simulink library "NCS_Library"  (R2019a)
settings: Solver=VariableStepAuto  StartTime=0.0  StopTime=10.0  RelTol=1e-3
values from neighbouring files (symbols this model uses):
  A = 10    [Parameter.m]
  band = 100000000    [Parameter.m]
  BER = 0    [Parameter.m]
  c = 5000000    [Parameter.m]
  c1 = 4.33    [Parameter.m]
  c2 = 3.16    [Parameter.m]
  CAN2EthernetDelay = 0.000    (= 0)    [Parameter.m]
  cR = 1.5*10^-3    (= 0.0015)    [Parameter.m]
  cw = (cwE * 2 + cwM * (nW_ges-2))/nW_ges    (= 0.1475)    [Parameter.m]
  cwE = 0.35    [Parameter.m]
  cwM = 0.08    [Parameter.m]
  Cycle_Controller = 0    [Parameter.m]
  CyclePLC = 24/1000    (= 0.024)    [Parameter.m]
  d = 800000    [Parameter.m]
  Dr = 0.92    [Parameter.m]
  Ethernet2CANDelay = 0.005    [Parameter.m]
  F_konst = 70892    [Parameter.m]
  FA = 100000    [Parameter.m]
  FB_WB_max = 10000    [Parameter.m]
  FBel_an = iG*nG*F_KZmax*nBan*R_mR/(Dr/2)    (= 28197.4297239)    [Parameter.m]
  FBel_frei = iG*nG*F_KZmax*nBfrei*R_mW/(Dr/2)    (= 29270.6882948)    [Parameter.m]
  Fmaxdyn = 300000    [Parameter.m]
  g = 9.81    [Parameter.m]
  i = 0    [Parameter.m]
  J = 1/2*mA*(Dr/2)^2    (= 158.7)    [Parameter.m]
  k1 = 0.095    [Parameter.m]
  k2 = 9.26/3.6    (= 2.57222222222)    [Parameter.m]
  k3 = 4.63/3.6    (= 1.28611111111)    [Parameter.m]
  mges = 58000    [Parameter.m]
  mu = [mu1 mu2]    [Parameter.m]
  muBel1 = 0.42    [Parameter.m]
  muBel2 = 0.36    [Parameter.m]
  n = 0.001    [Parameter.m]
  n_Mg = 4    [Parameter.m]
  n_WB = 4    [Parameter.m]
  nA = 4    [Parameter.m]
  nBan = 2    [Parameter.m]
  nBfrei = 3    [Parameter.m]
  nM = 4    [Parameter.m]
  nW_an = 4    [Parameter.m]
  P_max = 8200000    [Parameter.m]
  Q = 10    [Parameter.m]
  r_reib = 600    [Parameter.m]
  rho = 1.08    [Parameter.m]
  rhoL = 1.225    [Parameter.m]
  Size = 8    [Parameter.m]
  slip = [s1 s2]    [Parameter.m]
  tol = 0.05    [Parameter.m]
  v00 = 100/3.6    (= 27.7777777778)    [Parameter.m]
  v_grenz = 60/3.6    (= 16.6666666667)    [Parameter.m]
  v_opt = 75/3.6    (= 20.8333333333)    [Parameter.m]
  W_opt = 0.5    [Parameter.m]
  WB = 1    [Parameter.m]
  y_opt = sqrt(W_opt)/((1+sqrt(W_opt))^2+W_opt)    [Parameter.m]
undefined symbols (not defined in the file or in its folder): BUSCapacity, CableLength, controlGate, D_dyn, D_mg, EnableBurst, EnableToF, entity, Entity_out, Gate, Gate_4, Gate_5, Gate_ACK, Gate_copy, Gate_RX, getData, gettime, I_dyn, I_mg, m, magnitude, P_dyn, P_mg, ReadAttributes, readdata, ReadData, ReadSize, sigbuilder_block, Timeout, ToB, ToF, v0, v_d, v_soll
libraries: simulink x176, $bdroot x102
(part 6 of 12)

== system NCS_Library/Network/ETB/Burst Device/Protocl Stack ==
  Signal : Inport
  Parameter : Inport  Port=2
  RxFromBus : Inport  Port=3
  Bus Creator1 : BusCreator  Inputs=13
  Bus Selector : BusSelector  OutputSignals=SDTv2,T_Tx,msgType
  CycleRx : EntityServer  InputPortMessageModes=m  OutputPortMessageModes=m  Capacity=inf  ServiceTimeValue=CycleRx
  CycleTx : EntityServer  InputPortMessageModes=m  OutputPortMessageModes=m  Capacity=inf  ServiceTimeValue=CycleTx
  Data Type Conversion{,1..6} (7 alike) : DataTypeConversion  OutDataTypeStr=double
  Detect Change : simulink/Logic and Bit Operations/Detect Change  vinit=0  OutDataTypeStr=boolean
  IP : $bdroot/Network/ETB/OSI Layers/IP  SystemSampleTime=-1
  MAC Controller : $bdroot/Network/ETB/OSI Layers/MAC Controller  SystemSampleTime=-1
  Multiply : Product
  SDTv2 : $bdroot/Network/ETB/OSI Layers/SDTv2  SystemSampleTime=-1
  TRDP PD : Subsystem
  TRDP Timeout : $bdroot/Network/ETB/OSI Layers/TRDP Timeout  SystemSampleTime=-1
  UDP Single-Port : $bdroot/Network/ETB/OSI Layers/UDP Single-Port  SystemSampleTime=-1
  Data : Outport
  Recorder : Outport  Port=2
  TxToBus : Outport  Port=3
  wires:
  TRDP Timeout/1 -> [Valid]
  [Valid] -> Multiply/1
  SDTv2/1 -> Multiply/2  "Data"
  Multiply/1 -> Bus Creator1/2, Data/1
  CycleTx/1 -> MAC Controller/1
  IP/4 -> CycleTx/1
  MAC Controller/1 -> CycleRx/1
  CycleRx/1 -> IP/3
  IP/3 -> Bus Creator1/10  "delay"
  IP/2 -> Data Type Conversion5/1
  TRDP PD/6(msgType_receive) -> Data Type Conversion2/1
  TRDP PD/5(#Receive) -> Data Type Conversion6/1, TRDP Timeout/1
  TRDP PD/4(msgType_transmit) -> Data Type Conversion/1
  TRDP PD/3(#Transmit) -> Data Type Conversion1/1
  SDTv2/3 -> Bus Creator1/4  "Phase"
  SDTv2/2 -> Data Type Conversion3/1
  [SDTv2] -> Bus Creator1/13  "SDTv2"
  RxFromBus/1 -> MAC Controller/3
  UDP Single-Port/2 -> IP/1
  IP/1 -> UDP Single-Port/2
  UDP Single-Port/1 -> TRDP PD/3(InFromUDP)
  MAC Controller/2 -> Bus Creator1/11  "#collision"
  Signal/1 -> Bus Creator1/1, SDTv2/1  "Signal"
  Parameter/1 -> Bus Selector/1, IP/2, MAC Controller/2, TRDP PD/2(Paramter)
  Data Type Conversion/1 -> Bus Creator1/6  "msgType_transmit"
  Bus Creator1/1 -> Recorder/1
  TRDP PD/7(OutToUDP) -> UDP Single-Port/1
  SDTv2/4 -> TRDP PD/1(InFromSDTv2)
  TRDP PD/2(TRM) -> SDTv2/6
  Bus Selector/2 -> SDTv2/3  "<T_Tx>"
  TRDP PD/1(OutToSDTv2) -> SDTv2/5
  Bus Selector/3 -> SDTv2/4  "<msgType>"
  MAC Controller/4 -> TxToBus/1
  MAC Controller/3 -> Detect Change/1  "Retry"
  Detect Change/1 -> Data Type Conversion4/1
  Bus Selector/1 -> [SDTv2], SDTv2/2  "<SDTv2>"
  Data Type Conversion1/1 -> Bus Creator1/5  "#Transmit"
  Data Type Conversion2/1 -> Bus Creator1/8  "msgType_receive"
  Data Type Conversion3/1 -> Bus Creator1/3  "SSC"
  Data Type Conversion4/1 -> Bus Creator1/12  "Retry"
  Data Type Conversion5/1 -> Bus Creator1/9  "#damaged"
  Data Type Conversion6/1 -> Bus Creator1/7  "#Receive"

== system NCS_Library/Network/ETB/Burst Device/Subsystem ==
  In1 : Inport
  Entity Input Switch : EntityInputSwitch  InputPortMessageModes=m,m,m,m,m,m,m,m,m,m  OutputPortMessageModes=m  NumberInputPorts=10
      settings: InputPortMap=u1,u2,u3,u4,u5,u6,u7,u8,u9,u10
  Entity Replicator : EntityReplicator  InputPortMessageModes=m  OutputPortMessageModes=m,m,m,m,m,m,m,m,m,m  NumberReplicas=9
      settings: OutputPortMap=o0,o1,o2,o3,o4,o5,o6,o7,o8,o9
  Out1 : Outport
  wires:
  Entity Replicator/10 -> Entity Input Switch/10
  Entity Replicator/9 -> Entity Input Switch/9
  Entity Replicator/8 -> Entity Input Switch/8
  Entity Replicator/7 -> Entity Input Switch/7
  Entity Replicator/6 -> Entity Input Switch/6
  Entity Replicator/5 -> Entity Input Switch/5
  Entity Replicator/4 -> Entity Input Switch/4
  Entity Replicator/3 -> Entity Input Switch/3
  Entity Replicator/2 -> Entity Input Switch/2
  Entity Replicator/1 -> Entity Input Switch/1
  Entity Input Switch/1 -> Out1/1
  In1/1 -> Entity Replicator/1

== system NCS_Library/Network/ETB/Burst Device/Subsystem1 ==
  In1 : Inport
  Constant : Constant  Value=0  OutDataTypeStr=uint16
  Constant1 : Constant  Value=0  OutDataTypeStr=uint16
  Mux : Mux  Inputs=3
  Out1 : Outport
  wires:
  Constant1/1 -> Mux/3
  Constant/1 -> Mux/2
  Mux/1 -> Out1/1
  In1/1 -> Mux/1

== system NCS_Library/Network/ETB/Burst Device/Subsystem2 ==
  In1 : Inport
  Constant : Constant  Value=0  OutDataTypeStr=uint16
  Constant1 : Constant  Value=0  OutDataTypeStr=uint16
  Display : Display
  Display1 : Display
  Mux : Mux  Inputs=3
  Out1 : Outport
  wires:
  In1/1 -> Display/1, Mux/1
  Mux/1 -> Display1/1, Out1/1
  Constant/1 -> Mux/2
  Constant1/1 -> Mux/3

== system NCS_Library/Network/ETB/Burst Device/Subsystem3 ==
  In1 : Inport
  Constant : Constant  Value=0  OutDataTypeStr=uint16
  Constant1 : Constant  Value=0  OutDataTypeStr=uint16
  Mux : Mux  Inputs=3
  Out1 : Outport
  wires:
  Constant1/1 -> Mux/3
  Constant/1 -> Mux/2
  Mux/1 -> Out1/1
  In1/1 -> Mux/1

== system NCS_Library/Network/ETB/Cable/Simulink Function ==
  Time : Inport
  BitError : TriggerPort  TriggerType=function-call  IsSimulinkFunction=on  FunctionName=BitError  FunctionVisibility=scoped  VariantControl=(inherit)
  Constant : Constant  Value=BER
  MATLAB Function : MATLAB Function  TreatAsAtomicUnit=on
  SubnetID1 : ArgIn  OutDataTypeStr=uint16  PortDimensions=[1 4]  ArgumentName=Source
  SEQ : ArgIn  Port=2  OutDataTypeStr=uint32  ArgumentName=SEQ
  CheckBit : ArgOut  DisableCoverage=on  OutDataTypeStr=uint8  ArgumentName=CheckBit
  wires:
  Constant/1 -> MATLAB Function/4(BER)
  Time/1 -> MATLAB Function/1(Time)
  SEQ/1 -> MATLAB Function/3(SEQ)
  MATLAB Function/1(CheckBit) -> CheckBit/1
  SubnetID1/1 -> MATLAB Function/2(Source)

== system NCS_Library/Network/ETB/Controller Interface/Parameter ==
  note: User defined Parameters
  Add : Sum  Inputs=+-
  Bus Creator : BusCreator  Inputs=8
  Constant : Constant  Value=Address  OutDataTypeStr=uint16
  Constant1 : Constant  Value=Actuators  OutDataTypeStr=uint16
  Constant10 : Constant  Value=msgType_2  OutDataTypeStr=uint16
  Constant11 : Constant  Value=msgType_3  OutDataTypeStr=uint16
  Constant12 : Constant  Value=msgType_4  OutDataTypeStr=uint16
  Constant13 : Constant  Value=SDTv2_2
  Constant14 : Constant  Value=SDTv2_3
  Constant15 : Constant  Value=SDTv2_4
  Constant16 : Constant  Value=[0 0 0 0]  OutDataTypeStr=uint16
  Constant2 : Constant  Value=Tx_1  OutDataTypeStr=double
  Constant3 : Constant  Value=msgType_1  OutDataTypeStr=uint16
  Constant4 : Constant  Value=SDTv2_1
  Constant5 : Constant
  Constant6 : Constant  OutDataTypeStr=uint16
  Constant7 : Constant  Value=Tx_2  OutDataTypeStr=double
  Constant8 : Constant  Value=Tx_3  OutDataTypeStr=double
  Constant9 : Constant  Value=Tx_4  OutDataTypeStr=double
  MATLAB Function : MATLAB Function  TreatAsAtomicUnit=on
  MATLAB Function1 : MATLAB Function  TreatAsAtomicUnit=on
  Mux : Mux
  Mux1 : Mux
  Subscribe : Constant  Value=Sensors  OutDataTypeStr=uint16
  Subsystem1 : $bdroot/Network/ETB/ED/User Interface/Subsystem2  SystemSampleTime=-1
  Out1 : Outport
  wires:
  Constant6/1 -> Bus Creator/5  "Port"
  Constant7/1 -> Mux/2
  Constant8/1 -> Mux/3
  Constant1/1 -> MATLAB Function1/1(Actuators)
  MATLAB Function1/2(Subscribe) -> Bus Creator/3  "Subscribe"
  Constant16/1 -> Bus Creator/4  "ReplyAddress"
  Constant5/1 -> Add/2
  Constant2/1 -> Mux/1
  Constant3/1 -> MATLAB Function/1(In1)
  Constant12/1 -> MATLAB Function/4(In4)
  Constant9/1 -> Mux/4
  Constant10/1 -> MATLAB Function/2(In2)
  Constant4/1 -> Mux1/1
  Constant11/1 -> MATLAB Function/3(In3)
  Constant13/1 -> Mux1/2
  Mux1/1 -> Add/1
  Constant14/1 -> Mux1/3
  Mux/1 -> Bus Creator/6  "T_Tx"
  Add/1 -> Bus Creator/8  "SDTv2"
  MATLAB Function/1(msgType) -> Bus Creator/7  "msgType"
  Subscribe/1 -> MATLAB Function1/2(Sensors)
  Constant15/1 -> Mux1/4
  Bus Creator/1 -> Out1/1
  MATLAB Function1/1(Destination) -> Bus Creator/2  "Destination"
  Constant/1 -> Subsystem1/1  "Address"
  Subsystem1/1 -> Bus Creator/1  "Address"

== system NCS_Library/Network/ETB/Controller Interface/Subsystem ==
  InFromController : Inport
  Parameter : Inport  Port=2
  RxFromBus : Inport  Port=3
  Application1 : $bdroot/Network/ETB/OSI Layers/Application  Port=1
  Application2 : $bdroot/Network/ETB/OSI Layers/Application  Port=2
  Application3 : $bdroot/Network/ETB/OSI Layers/Application  Port=3
  Application4 : $bdroot/Network/ETB/OSI Layers/Application  Port=4
  Bus Creator : BusCreator  Inputs=2
  Data Type Conversion : DataTypeConversion  OutDataTypeStr=double
  Mux Y_M : MATLAB Function  TreatAsAtomicUnit=on
  Parameter{1..4} (4 alike) : InportShadow  Port=2
  Transport Layers : Subsystem
  OutToController : Outport
  Recorder : Outport  Port=2
  TxToBus : Outport  Port=3
  wires:
  Parameter/1 -> Transport Layers/5(Parameter)
  RxFromBus/1 -> Transport Layers/6(RxFromBus)
  Transport Layers/7(TxToBus) -> TxToBus/1
  Parameter1/1 -> Application1/2
  Mux Y_M/1(Y_M) -> OutToController/1  "Y_M"
  Parameter2/1 -> Application2/2
  Parameter3/1 -> Application3/2
  Parameter4/1 -> Application4/2
  InFromController/1 -> Application1/1, Application2/1, Application4/1, Application3/1  "u_4"
  Application1/1 -> Mux Y_M/1(in1)  "y_M_1"
  Application2/1 -> Mux Y_M/2(in2)  "y_M_2"
  Application3/1 -> Mux Y_M/3(in3)  "y_M_3"
  Application4/1 -> Mux Y_M/4(in4)  "y_M_4"
  Transport Layers/1(OutToApplication4) -> Application4/3
  Application4/2 -> Transport Layers/1(InFromApplication4)
  Transport Layers/2(OutToApplication3) -> Application3/3
  Application3/2 -> Transport Layers/2(InFromApplication3)
  Transport Layers/3(OutToApplication2) -> Application2/3
  Application2/2 -> Transport Layers/3(InFromApplication2)
  Transport Layers/4(OutToApplication1) -> Application1/3
  Application1/2 -> Transport Layers/4(InFromApplication1)
  Transport Layers/5(Delay) -> Bus Creator/1  "Delay"
  Data Type Conversion/1 -> Bus Creator/2  "#damaged"
  Bus Creator/1 -> Recorder/1
  Transport Layers/6(#damaged) -> Data Type Conversion/1

== system NCS_Library/Network/ETB/ED/Protocol Stack ==
  Signal : Inport
  Parameter : Inport  Port=2
  RxFromBus : Inport  Port=3
  Bus Selector : BusSelector  OutputSignals=SDTv2,T_Tx,msgType
  CycleRx : EntityServer  InputPortMessageModes=m  OutputPortMessageModes=m  Capacity=inf  ServiceTimeValue=CycleRx
  CycleTx : EntityServer  InputPortMessageModes=m  OutputPortMessageModes=m  Capacity=inf  ServiceTimeValue=CycleTx  EntryAction=ReadSize(entity.Size);
  Display : Display
  IP : $bdroot/Network/ETB/OSI Layers/IP  SystemSampleTime=-1
  MAC Controller : $bdroot/Network/ETB/OSI Layers/MAC Controller  SystemSampleTime=-1
  Multiply : Product
  SDTv2 : $bdroot/Network/ETB/OSI Layers/SDTv2  SystemSampleTime=-1
  Signal1 : InportShadow
  Simulink Function : Subsystem  TreatAsAtomicUnit=on
  Subsystem : Subsystem
  TRDP PD : $bdroot/Network/ETB/OSI Layers/TRDP PD  SystemSampleTime=-1
  TRDP Timeout : $bdroot/Network/Applications/TRDP Timeout  SystemSampleTime=-1
  UDP Single-Port : $bdroot/Network/ETB/OSI Layers/UDP Single-Port  SystemSampleTime=-1
  Data : Outport
  Recorder : Outport  Port=2
  TxToBus : Outport  Port=3
  wires:
  Bus Selector/1 -> [SDTv2], SDTv2/2  "<SDTv2>"
  MAC Controller/4 -> TxToBus/1
  Bus Selector/3 -> SDTv2/4  "<msgType>"
  TRDP PD/1 -> SDTv2/5
  Bus Selector/2 -> SDTv2/3  "<T_Tx>"
  TRDP PD/2 -> SDTv2/6
  SDTv2/4 -> TRDP PD/1
  TRDP PD/7 -> UDP Single-Port/1
  Parameter/1 -> TRDP PD/3, MAC Controller/2, IP/2, Bus Selector/1
  Signal/1 -> SDTv2/1, Subsystem/1(Signal)  "Signal"
  UDP Single-Port/1 -> TRDP PD/4
  IP/1 -> UDP Single-Port/2
  UDP Single-Port/2 -> IP/1
  RxFromBus/1 -> MAC Controller/3
  CycleRx/1 -> IP/3
  MAC Controller/1 -> CycleRx/1
  IP/4 -> CycleTx/1
  CycleTx/1 -> MAC Controller/1
  Signal1/1 -> TRDP PD/2  "Signal"
  Multiply/1 -> Subsystem/2(Data), Data/1  "Data"
  SDTv2/1 -> Multiply/2  "Data"
  [Valid] -> Multiply/1
  SDTv2/2 -> Subsystem/3(In3)
  SDTv2/3 -> Subsystem/4(Phase)  "Phase"
  TRDP PD/3 -> Subsystem/5(In5)
  TRDP PD/4 -> Subsystem/6(In6)
  TRDP PD/5 -> TRDP Timeout/1, Subsystem/7(In7)
  TRDP PD/6 -> Subsystem/8(In8)
  IP/2 -> Subsystem/9(In9)
  IP/3 -> Subsystem/10(delay)  "delay"
  MAC Controller/2 -> Subsystem/11(#collision)  "#collision"
  MAC Controller/3 -> Subsystem/12(Retry)  "Retry"
  Subsystem/1(Out1) -> Recorder/1
  [SDTv2] -> Subsystem/13(SDTv2)  "SDTv2"
  TRDP Timeout/1 -> [Valid]
  Simulink Function/1(Out1) -> Display/1

== system NCS_Library/Network/ETB/ED/User Interface ==
  note: User defined Parameters
  Add : Sum  Inputs=+-
  Bus Creator : BusCreator  Inputs=8
  Constant : Constant  Value=Address  OutDataTypeStr=uint16
  Constant1 : Constant  Value=Destination  OutDataTypeStr=uint16
  Constant2 : Constant  Value=Tx  OutDataTypeStr=double
  Constant3 : Constant  Value=msgType  OutDataTypeStr=uint8
  Constant4 : Constant  Value=SDTv2  OutDataTypeStr=double
  Constant5 : Constant
  Constant6 : Constant  Value=Port  OutDataTypeStr=uint16
  Constant7 : Constant  Value=ReplyAddress  OutDataTypeStr=uint16
  MATLAB Function : MATLAB Function  TreatAsAtomicUnit=on
  MATLAB Function1 : MATLAB Function  TreatAsAtomicUnit=on
  Subscribe : Constant  Value=Subscribe  OutDataTypeStr=uint16
  Subsystem1 : $bdroot/Network/ETB/ED/User Interface/Subsystem2  SystemSampleTime=-1
  Subsystem2 : Subsystem
  Subsystem3 : $bdroot/Network/ETB/ED/User Interface/Subsystem2  SystemSampleTime=-1
  Parameter : Outport
  wires:
  Constant2/1 -> Bus Creator/6  "T_Tx"
  Constant3/1 -> MATLAB Function/1(u)
  MATLAB Function/1(msgType) -> Bus Creator/7  "msgType"
  Constant/1 -> Subsystem1/1
  Subsystem2/1(Out1) -> Bus Creator/2  "Destination"
  Constant7/1 -> Subsystem3/1
  Constant6/1 -> Bus Creator/5  "Port"
  Constant1/1 -> Subsystem2/1(In1)
  Subscribe/1 -> MATLAB Function1/1(u)
  Constant5/1 -> Add/2
  Constant4/1 -> Add/1
  Add/1 -> Bus Creator/8  "SDTv2"
  MATLAB Function1/1(y) -> Bus Creator/3  "Subscribe"
  Bus Creator/1 -> Parameter/1
  Subsystem1/1 -> Bus Creator/1  "Address"
  Subsystem3/1 -> Bus Creator/4  "ReplyAddress"

== system NCS_Library/Network/ETB/Ethernet_2-port_Switch/Buffer_fill Control ==
  In1 : Inport
  Compare To Constant : simulink/Logic and Bit Operations/Compare To Constant  relop=>=  const=floor(buffer_size/(2*1500))  OutDataTypeStr=boolean
  Constant : Constant
  Message Send : MessageSend  OutputPortMessageModes=m
      settings: InputPortMap=u1
  Sum : Sum  Inputs=|++
  Out1 : Outport
  wires:
  Message Send/1 -> Out1/1
  Sum/1 -> Message Send/1
  Constant/1 -> Sum/2
  Compare To Constant/1 -> Sum/1
  In1/1 -> Compare To Constant/1

== system NCS_Library/Network/ETB/Ethernet_2-port_Switch/Buffer_fill Control1 ==
  In1 : Inport
  Compare To Constant : simulink/Logic and Bit Operations/Compare To Constant  relop=>=  const=floor(buffer_size/(2*1500))  OutDataTypeStr=boolean
  Constant : Constant
  Message Send : MessageSend  OutputPortMessageModes=m
      settings: InputPortMap=u1
  Sum : Sum  Inputs=|++
  Out1 : Outport
  wires:
  Message Send/1 -> Out1/1
  Sum/1 -> Message Send/1
  Constant/1 -> Sum/2
  Compare To Constant/1 -> Sum/1
  In1/1 -> Compare To Constant/1

== system NCS_Library/Network/ETB/Ethernet_2-port_Switch/Determine Port_L//R ==
  gate_s : TriggerPort  TriggerType=function-call  IsSimulinkFunction=on  FunctionName=gate_s  FunctionVisibility=scoped  VariantControl=(inherit)
  Add : Sum
  Constant : Constant
  Constant1 : Constant  Value=addstore
  Data Store Read : DataStoreRead  DataStoreName=N
  Data Store Read1 : DataStoreRead  DataStoreName=S
  Data Store Write : DataStoreWrite  DataStoreName=S
  Data Type Conversion : DataTypeConversion  OutDataTypeStr=uint8
  Gain : Gain  Gain=1/band
  MATLAB Function1 : MATLAB Function  TreatAsAtomicUnit=on
  t1 : ArgIn  DisableCoverage=on  OutDataTypeStr=uint16  ArgumentName=Destination
  f1 : ArgIn  Port=2  OutDataTypeStr=uint16  ArgumentName=Source
  s : ArgIn  Port=3  ArgumentName=Size
  gate : ArgOut  OutDataTypeStr=uint8  ArgumentName=gate
  time : ArgOut  Port=2  ArgumentName=time
  wires:
  Constant/1 -> Add/2
  Gain/1 -> time/1
  s/1 -> Gain/1
  t1/1 -> MATLAB Function1/1(Destination)
  f1/1 -> MATLAB Function1/2(Source)
  MATLAB Function1/1(Anew) -> Data Store Write/1
  Data Store Read1/1 -> MATLAB Function1/3(A)
  Data Store Read/1 -> MATLAB Function1/4(B)
  Constant1/1 -> MATLAB Function1/5(maxn)
  MATLAB Function1/2(y) -> Add/1
  Add/1 -> Data Type Conversion/1
  Data Type Conversion/1 -> gate/1

== system NCS_Library/Network/ETB/Ethernet_2-port_Switch/Determine Port_N ==
  gate_n : TriggerPort  TriggerType=function-call  IsSimulinkFunction=on  FunctionName=gate_n  FunctionVisibility=scoped  VariantControl=(inherit)
  Add : Sum
  Constant : Constant
  Constant1 : Constant  Value=addstore
  Data Store Read : DataStoreRead  DataStoreName=N
  Data Store Read1 : DataStoreRead  DataStoreName=S
  Data Store Write : DataStoreWrite  DataStoreName=N
  Data Type Conversion : DataTypeConversion  OutDataTypeStr=uint8
  Gain : Gain  Gain=1/band
  MATLAB Function : MATLAB Function  TreatAsAtomicUnit=on
  t : ArgIn  DisableCoverage=on  OutDataTypeStr=uint16  ArgumentName=Destination
  f : ArgIn  Port=2  OutDataTypeStr=uint16  ArgumentName=Source
  s1 : ArgIn  Port=3  ArgumentName=Size
  gate : ArgOut  OutDataTypeStr=uint8  ArgumentName=gate
  time : ArgOut  Port=2  ArgumentName=time
  wires:
  f/1 -> MATLAB Function/2(Source)
  s1/1 -> Gain/1
  t/1 -> MATLAB Function/1(Destination)
  Add/1 -> Data Type Conversion/1
  Gain/1 -> time/1
  Data Store Read1/1 -> MATLAB Function/4(B)
  Data Store Read/1 -> MATLAB Function/3(A)
  Constant1/1 -> MATLAB Function/5(maxn)
  MATLAB Function/2(y) -> Add/1
  Constant/1 -> Add/2
  MATLAB Function/1(Anew) -> Data Store Write/1
  Data Type Conversion/1 -> gate/1

== system NCS_Library/Network/ETB/Ethernet_3-port_switch/Buffer_fill Control ==
  In1 : Inport
  Compare To Constant : simulink/Logic and Bit Operations/Compare To Constant  relop=>=  const=floor(buffer_size/(3*1500))  OutDataTypeStr=boolean
  Constant : Constant
  Message Send : MessageSend  OutputPortMessageModes=m
      settings: InputPortMap=u1
  Sum : Sum  Inputs=|++
  Out1 : Outport
  wires:
  In1/1 -> Compare To Constant/1
  Compare To Constant/1 -> Sum/1
  Constant/1 -> Sum/2
  Sum/1 -> Message Send/1
  Message Send/1 -> Out1/1

== system NCS_Library/Network/ETB/Ethernet_3-port_switch/Buffer_fill Control1 ==
  In1 : Inport
  Compare To Constant : simulink/Logic and Bit Operations/Compare To Constant  relop=>=  const=floor(buffer_size/(3*1500))  OutDataTypeStr=boolean
  Constant : Constant
  Message Send : MessageSend  OutputPortMessageModes=m
      settings: InputPortMap=u1
  Sum : Sum  Inputs=|++
  Out1 : Outport
  wires:
  In1/1 -> Compare To Constant/1
  Compare To Constant/1 -> Sum/1
  Constant/1 -> Sum/2
  Sum/1 -> Message Send/1
  Message Send/1 -> Out1/1

== system NCS_Library/Network/ETB/Ethernet_3-port_switch/Buffer_fill Control2 ==
  In1 : Inport
  Compare To Constant : simulink/Logic and Bit Operations/Compare To Constant  relop=>=  const=floor(buffer_size/(3*1500))  OutDataTypeStr=boolean
  Constant : Constant
  Message Send : MessageSend  OutputPortMessageModes=m
      settings: InputPortMap=u1
  Sum : Sum  Inputs=|++
  Out1 : Outport
  wires:
  In1/1 -> Compare To Constant/1
  Compare To Constant/1 -> Sum/1
  Constant/1 -> Sum/2
  Sum/1 -> Message Send/1
  Message Send/1 -> Out1/1

== system NCS_Library/Network/ETB/Ethernet_3-port_switch/Determine Port_L ==
  gate_l : TriggerPort  TriggerType=function-call  IsSimulinkFunction=on  FunctionName=gate_l  FunctionVisibility=scoped  VariantControl=(inherit)
  Add : Sum
  Constant : Constant
  Constant1 : Constant  Value=addstore
  Data Store Read : DataStoreRead  DataStoreName=N
  Data Store Read1 : DataStoreRead  DataStoreName=L
  Data Store Read2 : DataStoreRead  DataStoreName=R
  Data Store Write : DataStoreWrite  DataStoreName=L
  Data Type Conversion : DataTypeConversion  OutDataTypeStr=uint8
  Gain : Gain  Gain=1/band
  MATLAB Function : MATLAB Function  TreatAsAtomicUnit=on
  t~ : ArgIn  OutDataTypeStr=uint16  ArgumentName=Destination
  f~ : ArgIn  DisableCoverage=on  Port=2  OutDataTypeStr=uint16  ArgumentName=Source
  s : ArgIn  Port=3  ArgumentName=Size
  gate : ArgOut  OutDataTypeStr=uint8  ArgumentName=gate
  time : ArgOut  Port=2  ArgumentName=time
  wires:
  Gain/1 -> time/1
  Add/1 -> Data Type Conversion/1
  Constant/1 -> Add/2
  s/1 -> Gain/1
  MATLAB Function/1(Anew) -> Data Store Write/1
  MATLAB Function/2(y) -> Add/1
  t~/1 -> MATLAB Function/1(Destination)
  f~/1 -> MATLAB Function/2(Source)
  Data Store Read1/1 -> MATLAB Function/3(A)
  Data Store Read/1 -> MATLAB Function/4(B)
  Data Store Read2/1 -> MATLAB Function/5(C)
  Constant1/1 -> MATLAB Function/6(maxn)
  Data Type Conversion/1 -> gate/1

== system NCS_Library/Network/ETB/Ethernet_3-port_switch/Determine Port_N ==
  gate_n : TriggerPort  TriggerType=function-call  IsSimulinkFunction=on  FunctionName=gate_n  FunctionVisibility=scoped  VariantControl=(inherit)
  Add : Sum
  Constant : Constant
  Constant1 : Constant  Value=addstore
  Data Store Read : DataStoreRead  DataStoreName=N
  Data Store Read1 : DataStoreRead  DataStoreName=L
  Data Store Read2 : DataStoreRead  DataStoreName=R
  Data Store Write : DataStoreWrite  DataStoreName=N
  Data Type Conversion : DataTypeConversion  OutDataTypeStr=uint8
  Gain : Gain  Gain=1/band
  MATLAB Function : MATLAB Function  TreatAsAtomicUnit=on
  Destination : ArgIn  OutDataTypeStr=uint16  ArgumentName=Destination
  Source : ArgIn  DisableCoverage=on  Port=2  OutDataTypeStr=uint16  ArgumentName=Source
  Size : ArgIn  Port=3  ArgumentName=Size
  gate : ArgOut  OutDataTypeStr=uint8  ArgumentName=gate
  time : ArgOut  Port=2  ArgumentName=time
  wires:
  Constant/1 -> Add/2
  Gain/1 -> time/1
  Constant1/1 -> MATLAB Function/6(maxn)
  MATLAB Function/1(Anew) -> Data Store Write/1
  MATLAB Function/2(y) -> Add/1
  Data Store Read/1 -> MATLAB Function/3(A)
  Source/1 -> MATLAB Function/2(Source)
  Destination/1 -> MATLAB Function/1(Destination)
  Size/1 -> Gain/1
  Add/1 -> Data Type Conversion/1
  Data Type Conversion/1 -> gate/1
  Data Store Read1/1 -> MATLAB Function/4(B)
  Data Store Read2/1 -> MATLAB Function/5(C)

== system NCS_Library/Network/ETB/Ethernet_3-port_switch/Determine Port_R ==
  gate_r : TriggerPort  TriggerType=function-call  IsSimulinkFunction=on  FunctionName=gate_r  FunctionVisibility=scoped  VariantControl=(inherit)
  Add : Sum
  Constant : Constant
  Constant1 : Constant  Value=addstore
  Data Store Read : DataStoreRead  DataStoreName=N
  Data Store Read1 : DataStoreRead  DataStoreName=L
  Data Store Read2 : DataStoreRead  DataStoreName=R
  Data Store Write : DataStoreWrite  DataStoreName=R
  Data Type Conversion : DataTypeConversion  OutDataTypeStr=uint8
  Gain : Gain  Gain=1/band
  MATLAB Function : MATLAB Function  TreatAsAtomicUnit=on
  t~ : ArgIn  OutDataTypeStr=uint16  ArgumentName=Destination
  f~ : ArgIn  DisableCoverage=on  Port=2  OutDataTypeStr=uint16  ArgumentName=Source
  s : ArgIn  Port=3  ArgumentName=Size
  gate : ArgOut  OutDataTypeStr=uint8  ArgumentName=gate
  time : ArgOut  Port=2  ArgumentName=time
  wires:
  Constant/1 -> Add/2
  Gain/1 -> time/1
  Constant1/1 -> MATLAB Function/6(maxn)
  MATLAB Function/1(Anew) -> Data Store Write/1
  MATLAB Function/2(y) -> Add/1
  Data Store Read2/1 -> MATLAB Function/3(A)
  Data Store Read/1 -> MATLAB Function/4(B)
  Data Store Read1/1 -> MATLAB Function/5(C)
  f~/1 -> MATLAB Function/2(Source)
  t~/1 -> MATLAB Function/1(Destination)
  s/1 -> Gain/1
  Add/1 -> Data Type Conversion/1
  Data Type Conversion/1 -> gate/1

== system NCS_Library/Network/ETB/OSI Layers/Application ==
  InFromController : Inport
  Paramter : Inport  Port=2
  InFromUDP : Inport  Port=3
  Edit Paramter : Subsystem
  Entity Output Switch : EntityOutputSwitch  InputPortMessageModes=m  OutputPortMessageModes=m,m  SwitchingCriterion=From attribute  SwitchAttributeName=Route
  Entity Server : EntityServer  InputPortMessageModes=m  OutputPortMessageModes=m  Capacity=1  ServiceTimeValue=0  EntryAction=entity.Route = Sort(entity.msgType);
  Receive Sensor Data : Subsystem
  Simulink Function : Subsystem  TreatAsAtomicUnit=on
  Transmit Actuator Data : Subsystem
  UDP_Port : Constant  Value=Port  OutDataTypeStr=uint16
  OutToController : Outport
  OutToUDP : Outport  Port=2
  wires:
  UDP_Port/1 -> Edit Paramter/1(UDP_Port)
  Receive Sensor Data/1(OutToController) -> OutToController/1  "y_M"
  Paramter/1 -> Edit Paramter/2(Parameter)
  Edit Paramter/1(Parameter_edited) -> Receive Sensor Data/1(Parameter), Transmit Actuator Data/3(Parameter)
  InFromUDP/1 -> Entity Server/1
  Transmit Actuator Data/1(OutToUDP) -> OutToUDP/1
  InFromController/1 -> Transmit Actuator Data/1(InFromController)  "u"
  Entity Server/1 -> Entity Output Switch/1
  Entity Output Switch/1 -> Receive Sensor Data/2(InFromUDP)  "Push by Sensor"
  Entity Output Switch/2 -> Transmit Actuator Data/2(InFromUDP)  "Pull Request by Actuator"

== system NCS_Library/Network/ETB/OSI Layers/IP ==
  note: Get Delay
  note: Addressing
  note: Receive
  note: Transmit
  note: Check Sum
  InFromUDP : Inport
  Paramter : Inport  Port=2
  InFromMAC : Inport  Port=3
  Add : Sum  Inputs=+-
  Bus Selector : BusSelector  OutputSignals=Address,Subscribe
  Clock : Clock
  Detect Change2 : simulink/Logic and Bit Operations/Detect Change  vinit=0  OutDataTypeStr=boolean
  Display : Display
  Display1 : Display
  Entity Output Switch : EntityOutputSwitch  InputPortMessageModes=m  OutputPortMessageModes=m,m  SwitchingCriterion=From attribute  SwitchAttributeName=CheckBit
  Entity Output Switch1 : EntityOutputSwitch  InputPortMessageModes=m  OutputPortMessageModes=m,m  SwitchingCriterion=From attribute  SwitchAttributeName=Route
  Entity Server : EntityServer  InputPortMessageModes=m  OutputPortMessageModes=m  Capacity=1  ServiceTimeValue=0  EntryAction=[ entity.Timestamp, entity.MACDestination, entity.MACSource ] = SetAttributes(entity.Destination, entity.Source);
  Entity Server1 : EntityServer  InputPortMessageModes=m  OutputPortMessageModes=n,m  Capacity=1  ServiceTimeValue=0  EntryAction=|  NumberEntitiesDeparted=on
      | entity.Route = getAttributes(entity.Timestamp, entity.Source, entity.Destination);
      | entity.CheckBit = entity.CheckBit+uint8(1);
      settings: OutputPortMap=o0,o9
  Entity Server2 : EntityServer  InputPortMessageModes=m  OutputPortMessageModes=n,m  Capacity=1  ServiceTimeValue=0  NumberEntitiesDeparted=on
      settings: OutputPortMap=o0,o9
  Entity Terminator : EntityTerminator  InputPortMessageModes=m  NumberEntitiesArrived=on
      settings: OutputPortMap=o0
  Entity Terminator1 : EntityTerminator  InputPortMessageModes=m  NumberEntitiesArrived=on
      settings: OutputPortMap=o0
  Simulink Function : Subsystem  TreatAsAtomicUnit=on
  Simulink Function1 : Subsystem  TreatAsAtomicUnit=on
  Subsystem : Subsystem
  OutToUDP : Outport
  #damaged : Outport  Port=2
  DELAY : Outport  Port=3
  OutToMAC : Outport  Port=4
  wires:
  InFromUDP/1 -> Entity Server/1
  Entity Server/1 -> OutToMAC/1
  InFromMAC/1 -> Entity Server1/1
  Entity Output Switch/1 -> Entity Terminator/1
  Entity Terminator/1 -> #damaged/1
  Clock/1 -> Simulink Function/1(time), [Time]
  Simulink Function1/1(Timestamp) -> Add/2
  Detect Change2/1 -> Subsystem/Enable
  Subsystem/1(DELAY) -> DELAY/1
  Add/1 -> Subsystem/1(delay)
  [Time] -> Add/1
  Entity Output Switch1/2 -> Entity Terminator1/1
  Entity Server1/2 -> Entity Output Switch1/1
  Entity Output Switch1/1 -> Entity Output Switch/1
  Entity Output Switch/2 -> Entity Server2/1
  Entity Server2/2 -> OutToUDP/1
  Entity Server2/1 -> Detect Change2/1
  Entity Server1/1 -> Display/1
  Bus Selector/1 -> Simulink Function1/1(Address)  "<Address>"
  Bus Selector/2 -> Simulink Function1/2(SN)  "<Subscribe>"
  Paramter/1 -> Bus Selector/1
  Entity Terminator1/1 -> Display1/1
  Simulink Function1/2(Source) -> Subsystem/2(Source)
  Simulink Function1/3(Destination) -> Subsystem/3(Destination)

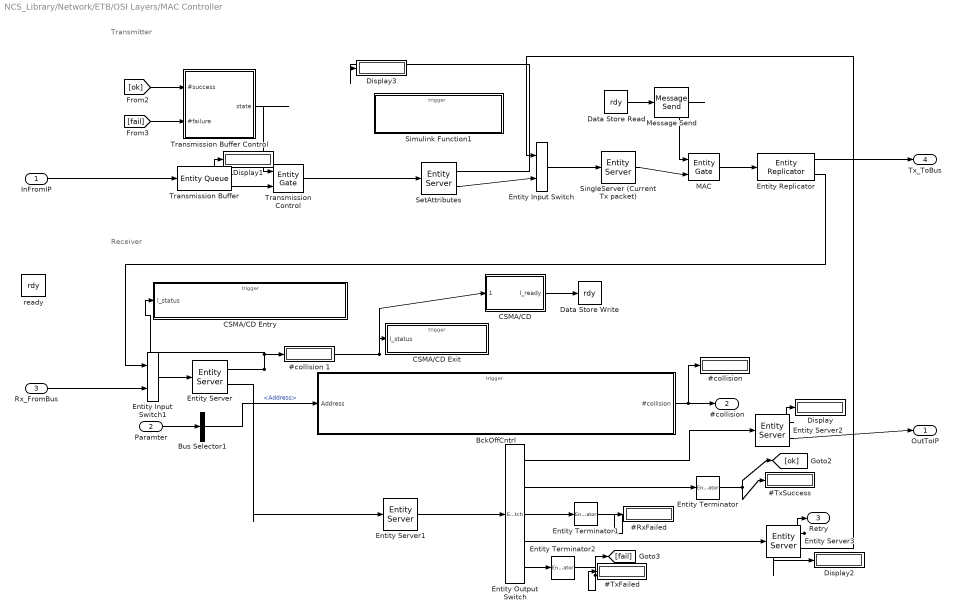
== system NCS_Library/Network/ETB/OSI Layers/MAC Controller ==
  note: Transmitter
  note: Receiver
  InFromIP : Inport
  Paramter : Inport  Port=2
  Rx_FromBus : Inport  Port=3
  #RxFailed : Display
  #TxFailed : Display
  #TxSuccess : Display
  "#collision " : Display
  #collision 1 : Display
  BckOffCntrl : Subsystem  TreatAsAtomicUnit=on
  Bus Selector1 : BusSelector  OutputSignals=Address
  CSMA/CD : Subsystem  TreatAsAtomicUnit=on
  CSMA/CD Entry : Subsystem  TreatAsAtomicUnit=on
  CSMA/CD Exit : Subsystem  TreatAsAtomicUnit=on
  Data Store Read : DataStoreRead  DataStoreName=rdy
  Data Store Write : DataStoreWrite  DataStoreName=rdy
  Display{,1..3} (4 alike) : Display
  Entity Input Switch : EntityInputSwitch  InputPortMessageModes=m,m  OutputPortMessageModes=m
  Entity Input Switch1 : EntityInputSwitch  InputPortMessageModes=m,m  OutputPortMessageModes=m
  Entity Output Switch : EntityOutputSwitch  InputPortMessageModes=m  OutputPortMessageModes=m,m,m,m,m  NumberOutputPorts=5  SwitchingCriterion=From attribute  SwitchAttributeName=Route
      settings: OutputPortMap=o0,o1,o2,o3,o4
  Entity Replicator : EntityReplicator  InputPortMessageModes=m  OutputPortMessageModes=m,m
  Entity Server : EntityServer  InputPortMessageModes=m  OutputPortMessageModes=n,m  Capacity=1000  ServiceTimeSource=Attribute  EntryAction=entity.ServiceTime = SetServiceTime(entity.Size);  NumberEntitiesInBlock=on
      settings: OutputPortMap=o1,o9
  Entity Server1 : EntityServer  InputPortMessageModes=m  OutputPortMessageModes=m  Capacity=1  ServiceTimeValue=0  EntryAction=[entity.Route,entity.NumCollision, entity.BckOffTime]=bckoffctrl(entity.NumCollision, entity.Collision, entity.MACSource, entity.MACDestination, entity.SEQ, entity.ServiceTime);
  Entity Server2 : EntityServer  InputPortMessageModes=m  OutputPortMessageModes=n,m  Capacity=1  ServiceTimeValue=0  NumberEntitiesDeparted=on
      settings: OutputPortMap=o0,o9
  Entity Server3 : EntityServer  InputPortMessageModes=m  OutputPortMessageModes=n,m  Capacity=1  ServiceTimeValue=0  NumberEntitiesDeparted=on
      settings: OutputPortMap=o0,o9
  Entity Terminator : EntityTerminator  InputPortMessageModes=m  NumberEntitiesArrived=on
      settings: OutputPortMap=o0
  Entity Terminator1 : EntityTerminator  InputPortMessageModes=m  NumberEntitiesArrived=on
      settings: OutputPortMap=o0
  Entity Terminator2 : EntityTerminator  InputPortMessageModes=m  NumberEntitiesArrived=on
      settings: OutputPortMap=o0
  MAC : EntityGate  InputPortMessageModes=m,m  OutputPortMessageModes=m
  Message Send : MessageSend  OutputPortMessageModes=m
      settings: InputPortMap=u1
  SetAttributes : EntityServer  InputPortMessageModes=m  OutputPortMessageModes=n,m  Capacity=1  ServiceTimeValue=0  EntryAction=|  NumberEntitiesDeparted=on
      | entity.ServiceTime = SetServiceTime(entity.Size);
      | % Init
      | entity.NumCollision=uint8(0);
      | entity.BckOffTime=0;
      settings: OutputPortMap=o0,o9
  Simulink Function1 : Subsystem  TreatAsAtomicUnit=on
  SingleServer (Current Tx packet) : EntityServer  InputPortMessageModes=m  OutputPortMessageModes=m  Capacity=1  ServiceTimeSource=Attribute  ServiceTimeValue=0  ServiceTimeAttributeName=BckOffTime  EntryAction=entity.Collision = uint8(0);
  Transmission Buffer : EntityQueue  InputPortMessageModes=m  OutputPortMessageModes=n,m  Capacity=100  NumberEntitiesInBlock=on
      settings: OutputPortMap=o1,o5
  Transmission Buffer Control : Subsystem
  Transmission Control : EntityGate  InputPortMessageModes=m,m  OutputPortMessageModes=m  OperatingMode=Release gate  OpenGateAtSimulationStart=on
  ready : DataStoreMemory  DataStoreName=rdy  ReadBeforeWriteMsg=warning  WriteAfterWriteMsg=warning  WriteAfterReadMsg=warning  InitialValue=1  ShowAdditionalParam=off
  OutToIP : Outport
  #collision : Outport  Port=2
  Retry : Outport  Port=3
  Tx_ToBus : Outport  Port=4
  wires:
  CSMA/CD/1(l_ready) -> Data Store Write/1
  Transmission Control/1 -> SetAttributes/1
  Entity Output Switch/2 -> Entity Terminator/1
  Data Store Read/1 -> Message Send/1
  Message Send/1 -> MAC/1
  Entity Output Switch/3 -> Entity Terminator1/1
  Entity Server1/1 -> Entity Output Switch/1
  SetAttributes/2 -> Entity Input Switch/2
  MAC/1 -> Entity Replicator/1
  Entity Input Switch1/1 -> Entity Server/1
  Entity Server/1 -> #collision 1/1, CSMA/CD Entry/1(l_status), CSMA/CD/1(l_status), CSMA/CD Exit/1(l_status)
  Entity Server/2 -> Entity Server1/1
  SingleServer (Current Tx packet)/1 -> MAC/2
  Entity Terminator1/1 -> #RxFailed/1
  Entity Input Switch/1 -> SingleServer (Current Tx packet)/1
  InFromIP/1 -> Transmission Buffer/1
  [ok] -> Transmission Buffer Control/1(#success)
  Transmission Buffer Control/1(state) -> Transmission Control/1
  [fail] -> Transmission Buffer Control/2(#failure)
  Transmission Buffer/2 -> Transmission Control/2
  Entity Output Switch/1 -> Entity Server2/1
  Entity Replicator/1 -> Tx_ToBus/1
  Entity Output Switch/5 -> Entity Terminator2/1
  Entity Replicator/2 -> Entity Input Switch1/1
  BckOffCntrl/1(#collision) -> #collision/1, "#collision "/1
  Rx_FromBus/1 -> Entity Input Switch1/2
  SetAttributes/1 -> Display3/1
  Paramter/1 -> Bus Selector1/1
  Bus Selector1/1 -> BckOffCntrl/1(Address)  "<Address>"
  Entity Server2/2 -> OutToIP/1
  Entity Terminator/1 -> [ok], #TxSuccess/1
  Entity Server2/1 -> Display/1
  Entity Output Switch/4 -> Entity Server3/1
  Entity Server3/2 -> Entity Input Switch/1
  Entity Server3/1 -> Retry/1, Display2/1
  Transmission Buffer/1 -> Display1/1
  Entity Terminator2/1 -> [fail], #TxFailed/1

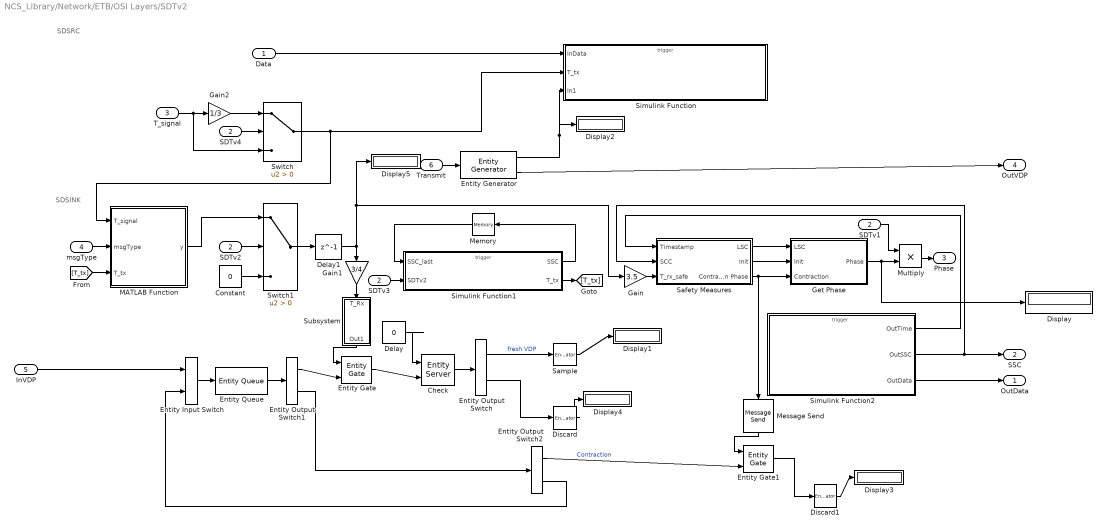
== system NCS_Library/Network/ETB/OSI Layers/SDTv2 ==
  note: SDSINK
  note: SDSRC
  Data : Inport
  SDTv2 : Inport  Port=2
  T_signal : Inport  Port=3
  msgType : Inport  Port=4
  InVDP : Inport  Port=5
  Transmit : Inport  Port=6
  Check : EntityServer  InputPortMessageModes=n,m  OutputPortMessageModes=m  Capacity=1  ServiceTimeSource=Signal port  ServiceTimeValue=0  EntryAction=[entity.Route] = Check(entity.SSC,entity.T_tx);
      settings: InputPortMap=u0,u2
  Constant : Constant  Value=0
  Delay : Constant  Value=0
  Delay1 : Delay  DelayLength=1
  Discard : EntityTerminator  InputPortMessageModes=m  NumberEntitiesArrived=on
      settings: OutputPortMap=o0
  Discard1 : EntityTerminator  InputPortMessageModes=m  NumberEntitiesArrived=on
      settings: OutputPortMap=o0
  Display{,1..5} (6 alike) : Display
  Entity Input Switch : EntityInputSwitch  InputPortMessageModes=m,m  OutputPortMessageModes=m
  Entity Output Switch : EntityOutputSwitch  InputPortMessageModes=m  OutputPortMessageModes=m,m  SwitchingCriterion=From attribute  SwitchAttributeName=Route
  Entity Output Switch1 : EntityOutputSwitch  InputPortMessageModes=m  OutputPortMessageModes=m,m  SwitchAttributeName=Attribute1
  Entity Output Switch2 : EntityOutputSwitch  InputPortMessageModes=m  OutputPortMessageModes=m,m  SwitchAttributeName=Attribute1
  Entity Gate : EntityGate  InputPortMessageModes=m,m  OutputPortMessageModes=m
  Entity Gate1 : EntityGate  InputPortMessageModes=m,m  OutputPortMessageModes=m  OpenGateAtSimulationStart=on
  Entity Generator : EntityGenerator  InputPortMessageModes=m  OutputPortMessageModes=n,m  GenerationMethod=Event-based  TimeSource=Signal port  GenerateAction=[ entity.SSC, entity.Data, entity.T_tx, entity.Size ] = SetAttributes();  NumberEntitiesDeparted=on  EntityType=Bus object  EntityTypeName=Ethernet_Entity
      settings: InputPortMap=u0  OutputPortMap=o0,o3
  Entity Queue : EntityQueue  InputPortMessageModes=m  OutputPortMessageModes=m
      settings: OutputPortMap=o5
  Gain : Gain  Gain=3.5
  Gain1 : Gain  Gain=3/4
  Gain2 : Gain  Gain=1/3
  Get Phase : Subsystem
  MATLAB Function : MATLAB Function  TreatAsAtomicUnit=on
  Memory : Memory  InheritSampleTime=on
  Message Send : MessageSend  OutputPortMessageModes=m
      settings: InputPortMap=u1
  Multiply : Product
  SDTv1 : InportShadow  Port=2
  SDTv3 : InportShadow  Port=2
  SDTv4 : InportShadow  Port=2
  Safety Measures : Subsystem
  Sample : EntityTerminator  InputPortMessageModes=m  EntryAction=ReadAttributes(entity.SSC, entity.Data, entity.Timestamp);  NumberEntitiesArrived=on
      settings: OutputPortMap=o0
  Simulink Function : Subsystem  TreatAsAtomicUnit=on
  Simulink Function1 : Subsystem  TreatAsAtomicUnit=on
  Simulink Function2 : Subsystem  TreatAsAtomicUnit=on
  Subsystem : Subsystem
  Switch : Switch  Criteria=u2 > Threshold
  Switch1 : Switch  Criteria=u2 > Threshold
  OutData : Outport
  SSC : Outport  Port=2
  Phase : Outport  Port=3
  OutVDP : Outport  Port=4
  wires:
  Entity Generator/1 -> Display2/1, Simulink Function/3(In1)
  Data/1 -> Simulink Function/1(InData)
  Check/1 -> Entity Output Switch/1
  Simulink Function1/1(SSC) -> Memory/1
  Memory/1 -> Simulink Function1/1(SSC_last)
  Sample/1 -> Display1/1
  Entity Gate/1 -> Check/2
  Subsystem/1(Out1) -> Entity Gate/1
  Gain1/1 -> Subsystem/1(T_Rx)
  Delay/1 -> Check/1
  Entity Output Switch1/1 -> Entity Gate/2
  Entity Queue/1 -> Entity Output Switch1/1
  Entity Input Switch/1 -> Entity Queue/1
  InVDP/1 -> Entity Input Switch/1
  Entity Output Switch1/2 -> Entity Output Switch2/1
  Entity Output Switch2/2 -> Entity Input Switch/2
  Entity Output Switch2/1 -> Entity Gate1/2  "Contraction"
  Message Send/1 -> Entity Gate1/1
  Entity Gate1/1 -> Discard1/1
  Discard1/1 -> Display3/1
  Discard/1 -> Display4/1
  Entity Output Switch/2 -> Discard/1
  Entity Output Switch/1 -> Sample/1  "fresh VDP"
  Safety Measures/3(Contraction Phase) -> Message Send/1, Get Phase/3(Contraction)
  Safety Measures/1(LSC) -> Get Phase/1(LSC)
  Safety Measures/2(Init) -> Get Phase/2(Init)
  Transmit/1 -> Entity Generator/1
  Simulink Function2/3(OutData) -> OutData/1
  Simulink Function2/2(OutSSC) -> Safety Measures/2(SCC), SSC/1
  Simulink Function1/2(T_tx) -> [T_tx]
  [T_tx] -> MATLAB Function/3(T_tx)
  msgType/1 -> MATLAB Function/2(msgType)
  Simulink Function2/1(OutTime) -> Safety Measures/1(Timestamp)
  Gain/1 -> Safety Measures/3(T_rx_safe)
  Entity Generator/2 -> OutVDP/1
  Delay1/1 -> Gain1/1, Display5/1, Gain/1
  Switch1/1 -> Delay1/1
  MATLAB Function/1(y) -> Switch1/1
  SDTv2/1 -> Switch1/2
  Constant/1 -> Switch1/3
  SDTv3/1 -> Simulink Function1/2(SDTv2)
  Get Phase/1(Phase) -> Display/1, Multiply/2
  Multiply/1 -> Phase/1
  SDTv1/1 -> Multiply/1
  SDTv4/1 -> Switch/2
  T_signal/1 -> Gain2/1, Switch/3
  Gain2/1 -> Switch/1
  Switch/1 -> MATLAB Function/1(T_signal), Simulink Function/2(T_tx)

== system NCS_Library/Network/ETB/OSI Layers/TRDP PD ==
  note: Receive
  note: Transmit
  InFromSDTv2 : Inport
  Data : Inport  Port=2
  Paramter : Inport  Port=3
  InFromUDP : Inport  Port=4
  Bus Selector : BusSelector  OutputSignals=T_Tx,SDTv2,msgType,Destination
  Bus Selector1 : BusSelector  OutputSignals=Address,Port,ReplyAddress
  Compare To Zero : simulink/Logic and Bit Operations/Compare To Zero  relop=>  OutDataTypeStr=boolean
  Compare To Zero1 : simulink/Logic and Bit Operations/Compare To Zero  relop=>  OutDataTypeStr=boolean
  Constant2 : Constant
  Delay : Delay  DelayLength=1
  Delay1 : Delay  DelayLength=1
  Detect Change : simulink/Logic and Bit Operations/Detect Change  vinit=0  OutDataTypeStr=boolean
  Detect Event : Subsystem
  Display : Display
  Display4 : Display
  Enabled Subsystem1 : Subsystem  TreatAsAtomicUnit=on
  Entity Server : EntityServer  InputPortMessageModes=m  OutputPortMessageModes=n,m  Capacity=1  ServiceTimeValue=0  EntryAction=ReadData( entity.msgType, entity.ReplyAddress, entity.Source);  NumberEntitiesDeparted=on
      settings: OutputPortMap=o0,o9
  Entity Server1 : EntityServer  InputPortMessageModes=m  OutputPortMessageModes=n,m  Capacity=1  ServiceTimeValue=0  EntryAction=[entity.SEQ, entity.msgType, entity.Destination, entity.Source, entity.CheckBit, entity.Data, entity.Port, entity.ReplyAddress] = SetAttributes(entity.SSC, entity.Data);  NumberEntitiesDeparted=on
      settings: OutputPortMap=o0,o9
  MATLAB Function1 : MATLAB Function  TreatAsAtomicUnit=on
  Memory2 : Memory  InheritSampleTime=on
  Memory3 : Memory  InheritSampleTime=on
  Message Send : MessageSend  OutputPortMessageModes=m  ShowEnablePort=on
      settings: InputPortMap=e0,u1
  Simulink Function : Subsystem  TreatAsAtomicUnit=on
  Simulink Function1 : Subsystem  TreatAsAtomicUnit=on
  Subsystem : Subsystem
  Transmit : MATLAB Function  TreatAsAtomicUnit=on
  OutToSDTv2 : Outport
  TRM : Outport  Port=2
  #Transmit : Outport  Port=3
  msgType_transmit : Outport  Port=4
  #Receive : Outport  Port=5
  msgType_receive : Outport  Port=6
  OutToUDP : Outport  Port=7
  wires:
  InFromUDP/1 -> Entity Server/1
  Memory2/1 -> Transmit/1(Buffer_old)
  Transmit/2(lst_old) -> Memory3/1
  Transmit/1(Buffer) -> Memory2/1
  Memory3/1 -> Transmit/2(lst)
  Bus Selector/1 -> Subsystem/1(T_signal), MATLAB Function1/3(T_tx)  "<T_Tx>"
  Bus Selector/4 -> Transmit/10(DestinationPush)  "<Destination>"
  MATLAB Function1/1(Push) -> Transmit/7(Push)
  Compare To Zero/1 -> Message Send/1, Display4/1
  Compare To Zero1/1 -> Transmit/3(Pull)
  Entity Server/2 -> OutToSDTv2/1
  Paramter/1 -> Bus Selector1/1, Bus Selector/1
  Entity Server1/2 -> OutToUDP/1
  InFromSDTv2/1 -> Entity Server1/1
  Enabled Subsystem1/1(msgTypeReply) -> Delay/1
  Enabled Subsystem1/2(DestinationReply) -> Delay1/1
  Simulink Function1/1(msgType) -> msgType_receive/1, Enabled Subsystem1/1(msgType)
  Simulink Function1/2(ReplyAddress) -> Enabled Subsystem1/2(ReplyAddress)
  Detect Change/1 -> Enabled Subsystem1/Enable
  Entity Server/1 -> #Receive/1, Detect Change/1
  Delay/1 -> Transmit/4(msgTypeReply), Compare To Zero1/1
  Delay1/1 -> Transmit/5(DestinationReply)
  Detect Event/1(Event) -> MATLAB Function1/1(Event)
  Transmit/4(Destination) -> Simulink Function/2(Destination)
  Entity Server1/1 -> #Transmit/1
  Data/1 -> Detect Event/1(Data)
  Subsystem/1(Out1) -> MATLAB Function1/2(Time), Transmit/6(Cycle)
  Bus Selector/3 -> Display/1, MATLAB Function1/4(msgType), Transmit/9(msgTypePush)  "<msgType>"
  Bus Selector/2 -> Transmit/8(SDTv2), Subsystem/2(SDTv2)  "<SDTv2>"
  Bus Selector1/1 -> Simulink Function/3(Source)  "<Address>"
  Bus Selector1/2 -> Simulink Function/4(UDP)  "<Port>"
  Bus Selector1/3 -> Simulink Function/5(ReplyAddress)  "<ReplyAddress>"
  Message Send/1 -> TRM/1
  Constant2/1 -> Message Send/2
  Transmit/3(msgType) -> msgType_transmit/1, Compare To Zero/1, Simulink Function/1(msgType)

== system NCS_Library/Network/ETB/OSI Layers/TRDP Timeout ==
  #Received : Inport
  Clock : Clock
  Constant : Constant  Value=Timeout
  Detect Change : simulink/Logic and Bit Operations/Detect Change  vinit=0  OutDataTypeStr=boolean
  Logical Operator : Logic  Operator=NOT  Inputs=1  AllPortsSameDT=off  OutDataTypeStr=boolean
  TRDP Timeout : Stateflow chart  TreatAsAtomicUnit=on
  Valid : Outport
  wires:
  #Received/1 -> Detect Change/1
  Detect Change/1 -> TRDP Timeout/1(Reception)
  Clock/1 -> TRDP Timeout/2(Clock)
  Constant/1 -> TRDP Timeout/3(Timeout_Value)
  TRDP Timeout/1(Timeout) -> Logical Operator/1
  Logical Operator/1 -> Valid/1

== system NCS_Library/Network/ETB/OSI Layers/UDP Multi-Port ==
  note: IP to TRDP
  note: TRDP to IP
  InFromTRDP1 : Inport
  InFromTRDP2 : Inport  Port=2
  InFromTRDP3 : Inport  Port=3
  InFromTRDP4 : Inport  Port=4
  InFromTRDP5 : Inport  Port=5
  InFromTRDP6 : Inport  Port=6
  InFromTRDP7 : Inport  Port=7
  InFromTRDP8 : Inport  Port=8
  InFromIP : Inport  Port=9
  Entity Input Switch : EntityInputSwitch  InputPortMessageModes=m,m,m,m,m,m,m,m  OutputPortMessageModes=m  NumberInputPorts=8
      settings: InputPortMap=u1,u2,u3,u4,u5,u6,u7,u8
  Entity Input Switch{1..8} (8 alike) : EntityInputSwitch  InputPortMessageModes=m,m  OutputPortMessageModes=m
  Entity Output Switch : EntityOutputSwitch  InputPortMessageModes=m  OutputPortMessageModes=m,m,m,m,m,m,m,m,m  NumberOutputPorts=9  SwitchingCriterion=From attribute  SwitchAttributeName=Port
      settings: OutputPortMap=o0,o1,o2,o3,o4,o5,o6,o7,o8
  Entity Replicator : EntityReplicator  InputPortMessageModes=m  OutputPortMessageModes=m,m,m,m,m,m,m,m,m  NumberReplicas=8
      settings: OutputPortMap=o0,o1,o2,o3,o4,o5,o6,o7,o8
  Entity Terminator : EntityTerminator  InputPortMessageModes=m
  OutToTRDP1 : Outport
  OutToTRDP2 : Outport  Port=2
  OutToTRDP3 : Outport  Port=3
  OutToTRDP4 : Outport  Port=4
  OutToTRDP5 : Outport  Port=5
  OutToTRDP6 : Outport  Port=6
  OutToTRDP7 : Outport  Port=7
  OutToTRDP8 : Outport  Port=8
  OutToIP : Outport  Port=9
  wires:
  InFromIP/1 -> Entity Output Switch/1
  Entity Input Switch/1 -> OutToIP/1
  InFromTRDP1/1 -> Entity Input Switch/1
  InFromTRDP8/1 -> Entity Input Switch/8
  InFromTRDP7/1 -> Entity Input Switch/7
  InFromTRDP6/1 -> Entity Input Switch/6
  InFromTRDP4/1 -> Entity Input Switch/4
  InFromTRDP3/1 -> Entity Input Switch/3
  InFromTRDP2/1 -> Entity Input Switch/2
  InFromTRDP5/1 -> Entity Input Switch/5
  Entity Output Switch/9 -> Entity Replicator/1  "Multicast"
  Entity Input Switch1/1 -> OutToTRDP1/1
  Entity Input Switch5/1 -> OutToTRDP5/1
  Entity Input Switch2/1 -> OutToTRDP2/1
  Entity Input Switch8/1 -> OutToTRDP8/1
  Entity Input Switch7/1 -> OutToTRDP7/1
  Entity Input Switch6/1 -> OutToTRDP6/1
  Entity Input Switch4/1 -> OutToTRDP4/1
  Entity Input Switch3/1 -> OutToTRDP3/1
  Entity Output Switch/1 -> Entity Input Switch1/1  "Port 1"
  Entity Output Switch/2 -> Entity Input Switch2/1  "Port 2"
  Entity Output Switch/3 -> Entity Input Switch3/1  "Port 3"
  Entity Output Switch/4 -> Entity Input Switch4/1  "Port 4"
  Entity Output Switch/5 -> Entity Input Switch5/1  "Port 5"
  Entity Output Switch/6 -> Entity Input Switch6/1  "Port 6"
  Entity Output Switch/7 -> Entity Input Switch7/1  "Port 7"
  Entity Output Switch/8 -> Entity Input Switch8/1  "Port 8"
  Entity Replicator/1 -> Entity Input Switch1/2
  Entity Replicator/2 -> Entity Input Switch2/2
  Entity Replicator/3 -> Entity Input Switch3/2
  Entity Replicator/4 -> Entity Input Switch4/2
  Entity Replicator/5 -> Entity Input Switch5/2
  Entity Replicator/6 -> Entity Input Switch6/2
  Entity Replicator/7 -> Entity Input Switch7/2
  Entity Replicator/8 -> Entity Input Switch8/2
  Entity Replicator/9 -> Entity Terminator/1

== system NCS_Library/Network/ETB/OSI Layers/UDP Single-Port ==
  note: Use this UDP layer for single port end devices for a better perfomance
  InFromTRDP : Inport
  InFromIP : Inport  Port=2
  OutToTRDP : Outport
  OutToIP : Outport  Port=2
  wires:
  InFromIP/1 -> OutToTRDP/1
  InFromTRDP/1 -> OutToIP/1
